simulink model "Advanced_Voter"  (R2018b)
settings: Solver=VariableStepAuto  StartTime=0.0  StopTime=10.0  RelTol=1e-3
settings Model: Creator=diepe  LastModifiedBy=diepe

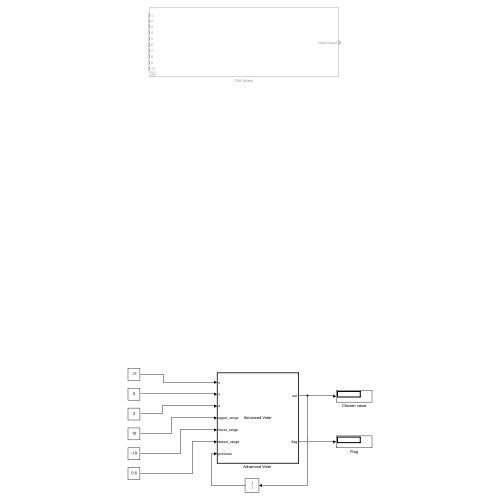
[thumbnail: Simulink's stored preview of the top-level diagram]
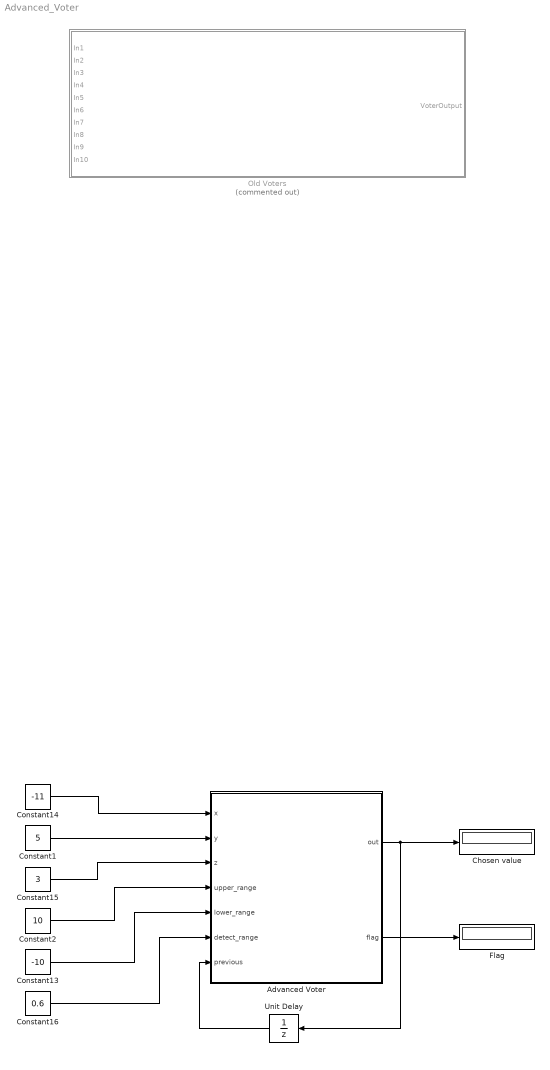
== system Advanced_Voter ==
  "Advanced Voter " : MATLAB Function  TreatAsAtomicUnit=on
  Chosen value : Display
  Constant1 : Constant  Value=5  OutDataTypeStr=double
  Constant13 : Constant  Value=-10  OutDataTypeStr=double
  Constant14 : Constant  Value=-11  OutDataTypeStr=double
  Constant15 : Constant  Value=3  OutDataTypeStr=double
  Constant16 : Constant  Value=0.6  OutDataTypeStr=double
  Constant2 : Constant  Value=10  OutDataTypeStr=double
  Flag : Display
  Old Voters : Subsystem  Commented=on
  Unit Delay : UnitDelay  SampleTime=-1  HasFrameUpgradeWarning=on
  wires:
  Unit Delay/1 -> "Advanced Voter "/7(previous)
  Constant2/1 -> "Advanced Voter "/4(upper_range)
  Constant14/1 -> "Advanced Voter "/1(x)
  Constant1/1 -> "Advanced Voter "/2(y)
  Constant13/1 -> "Advanced Voter "/5(lower_range)
  Constant15/1 -> "Advanced Voter "/3(z)
  Constant16/1 -> "Advanced Voter "/6(detect_range)
  "Advanced Voter "/2(flag) -> Flag/1
  "Advanced Voter "/1(out) -> Chosen value/1, Unit Delay/1

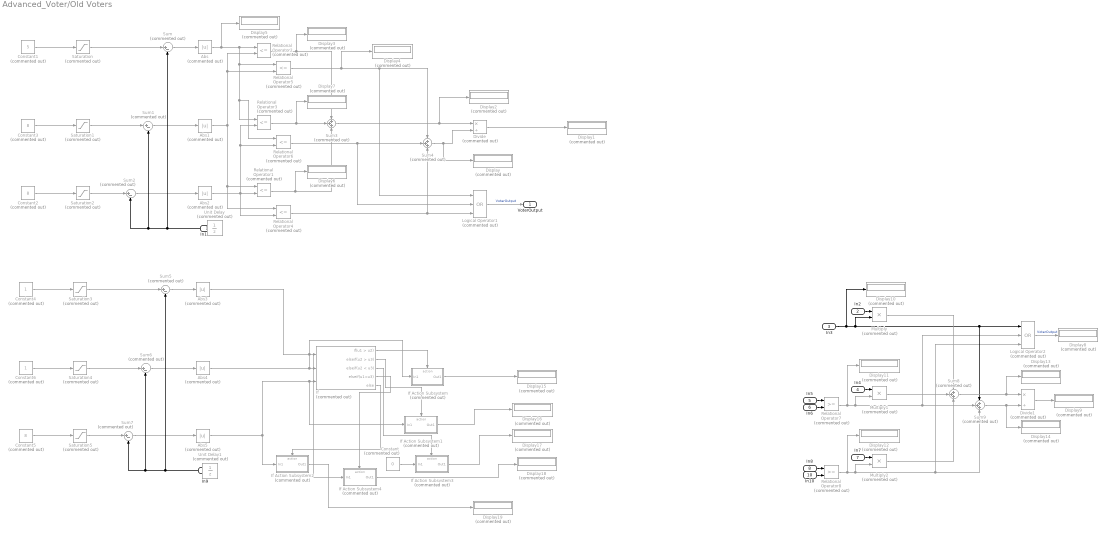
== system Advanced_Voter/Old Voters ==
  In1 : Inport
  In2 : Inport  Port=2
  In3 : Inport  Port=3
  In4 : Inport  Port=4
  In5 : Inport  Port=5
  In6 : Inport  Port=6
  In7 : Inport  Port=7
  In8 : Inport  Port=8
  In9 : Inport  Port=9
  In10 : Inport  Port=10
  Abs{,1..5} (6 alike) : Abs  Commented=on
  Constant : Constant  Commented=on  Value=0
  Constant1 : Constant  Commented=on  Value=5  OutDataTypeStr=int16
  Constant2 : Constant  Commented=on  Value=8  OutDataTypeStr=int16
  Constant3 : Constant  Commented=on  Value=8  OutDataTypeStr=int16
  Constant4 : Constant  Commented=on  OutDataTypeStr=int16
  Constant5 : Constant  Commented=on  Value=8  OutDataTypeStr=int16
  Constant6 : Constant  Commented=on  OutDataTypeStr=int16
  Display{,1..19} (20 alike) : Display  Commented=on
  Divide : Product  Commented=on  Inputs=*/
  Divide1 : Product  Commented=on  Inputs=*/
  If : If  Commented=on  NumInputs=3  IfExpression=u1 > u2  ElseIfExpressions=u2 > u3, u2 < u3, u1<u3
  If Action Subsystem : Subsystem  Commented=on  TreatAsAtomicUnit=on
  If Action Subsystem1 : Subsystem  Commented=on  TreatAsAtomicUnit=on
  If Action Subsystem2 : Subsystem  Commented=on  TreatAsAtomicUnit=on
  If Action Subsystem3 : Subsystem  Commented=on  TreatAsAtomicUnit=on
  If Action Subsystem4 : Subsystem  Commented=on  TreatAsAtomicUnit=on
  Logical Operator1 : Logic  Commented=on  Operator=OR  Inputs=3  AllPortsSameDT=off  OutDataTypeStr=boolean
  Logical Operator2 : Logic  Commented=on  Operator=OR  Inputs=3  AllPortsSameDT=off  OutDataTypeStr=boolean
  Multiply : Product  Commented=on
  Multiply1 : Product  Commented=on
  Multiply2 : Product  Commented=on
  Relational Operator1 : RelationalOperator  Commented=on  Operator=<=  RndMeth=Simplest
  Relational Operator{2,4..6} (4 alike) : RelationalOperator  Commented=on  Operator=<=  OutDataTypeStr=boolean  RndMeth=Simplest
  Relational Operator3 : RelationalOperator  Commented=on  Operator=<=  RndMeth=Simplest
  Relational Operator7 : RelationalOperator  Commented=on  OutDataTypeStr=boolean  RndMeth=Simplest
  Relational Operator8 : RelationalOperator  Commented=on  OutDataTypeStr=boolean  RndMeth=Simplest
  Saturation{,1..5} (6 alike) : Saturate  Commented=on  UpperLimit=10  LowerLimit=-10
  Sum{,1..2,5..7} (6 alike) : Sum  Commented=on  Inputs=|+-
  Sum{3..4,8..9} (4 alike) : Sum  Commented=on  Inputs=+++
  Unit Delay : UnitDelay  Commented=on  SampleTime=-1  HasFrameUpgradeWarning=on
  Unit Delay1 : UnitDelay  Commented=on  SampleTime=-1  HasFrameUpgradeWarning=on
  VoterOutput : Outport
  wires:
  Sum1/1 -> Abs1/1
  Abs3/1 -> If Action Subsystem4/1(In1), If/1
  Saturation/1 -> Sum/1
  Relational Operator8/1 -> Display12/1, Logical Operator2/3, Sum9/3, Multiply2/2
  Sum4/1 -> Display/1, Divide/2
  Relational Operator3/1 -> Display7/1, Sum3/2
  If Action Subsystem3/1(Out1) -> Display17/1
  Relational Operator7/1 -> Display11/1, Logical Operator2/2, Sum9/2, Multiply1/2
  Relational Operator1/1 -> Display6/1, Sum3/3
  Abs/1 -> Display5/1, Relational Operator5/1, Relational Operator6/1, Relational Operator3/1, Relational Operator2/1
  In3/1 -> Display10/1, Logical Operator2/1, Sum9/1, Multiply/2
  Relational Operator5/1 -> Display4/1, Sum4/1, Logical Operator1/1
  Abs1/1 -> Relational Operator4/1, Relational Operator1/1, Relational Operator5/2, Relational Operator2/2
  Sum5/1 -> Abs3/1
  Constant6/1 -> Saturation4/1
  Sum7/1 -> Abs5/1
  Sum9/1 -> Display14/1, Divide1/2
  Divide1/1 -> Display9/1
  Divide/1 -> Display1/1
  If Action Subsystem1/1(Out1) -> Display16/1
  Sum2/1 -> Abs2/1
  If/3 -> If Action Subsystem3/Action
  Saturation1/1 -> Sum1/1
  Sum/1 -> Abs/1
  Relational Operator2/1 -> Display3/1, Sum3/1
  Sum3/1 -> Display2/1, Divide/1
  Saturation4/1 -> Sum6/1
  Constant4/1 -> Saturation3/1
  Constant2/1 -> Saturation2/1
  If Action Subsystem4/1(Out1) -> Display18/1
  Constant3/1 -> Saturation1/1
  Abs4/1 -> If Action Subsystem/1(In1), If/2
  Relational Operator6/1 -> Sum4/2, Logical Operator1/2
  Sum6/1 -> Abs4/1
  In7/1 -> Multiply2/1
  Multiply/1 -> Sum8/1
  Saturation3/1 -> Sum5/1
  Multiply2/1 -> Sum8/3
  Abs2/1 -> Relational Operator6/2, Relational Operator3/2, Relational Operator4/2, Relational Operator1/2
  Sum8/1 -> Display13/1, Divide1/1
  In2/1 -> Multiply/1
  Constant5/1 -> Saturation5/1
  Logical Operator2/1 -> Display8/1  "VoterOutput"
  If/1 -> If Action Subsystem/Action
  If Action Subsystem2/1(Out1) -> Display19/1
  Saturation5/1 -> Sum7/1
  In1/1 -> Sum2/2, Sum1/2, Sum/2
  If/4 -> If Action Subsystem4/Action
  In8/1 -> Relational Operator8/1
  If/5 -> If Action Subsystem2/Action
  Multiply1/1 -> Sum8/2
  Abs5/1 -> If Action Subsystem2/1(In1), If Action Subsystem1/1(In1), If/3
  If Action Subsystem/1(Out1) -> Display15/1
  If/2 -> If Action Subsystem1/Action
  In9/1 -> Sum7/2, Sum6/2, Sum5/2
  Constant1/1 -> Saturation/1
  Constant/1 -> If Action Subsystem3/1(In1)
  In5/1 -> Relational Operator7/1
  Saturation2/1 -> Sum2/1
  Relational Operator4/1 -> Sum4/3, Logical Operator1/3
  In4/1 -> Multiply1/1
  Logical Operator1/1 -> VoterOutput/1  "VoterOutput"
  In10/1 -> Relational Operator8/2
  In6/1 -> Relational Operator7/2

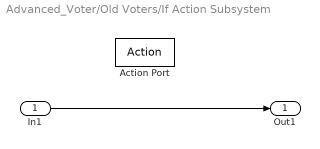
== system Advanced_Voter/Old Voters/If Action Subsystem ==
  In1 : Inport
  Action Port : ActionPort
  Out1 : Outport  VectorParamsAs1DForOutWhenUnconnected=off
  wires:
  In1/1 -> Out1/1

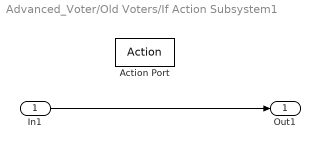
== system Advanced_Voter/Old Voters/If Action Subsystem1 ==
  In1 : Inport
  Action Port : ActionPort
  Out1 : Outport  VectorParamsAs1DForOutWhenUnconnected=off
  wires:
  In1/1 -> Out1/1

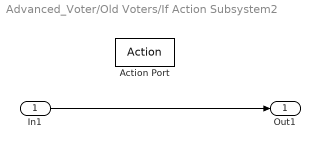
== system Advanced_Voter/Old Voters/If Action Subsystem2 ==
  In1 : Inport
  Action Port : ActionPort
  Out1 : Outport  VectorParamsAs1DForOutWhenUnconnected=off
  wires:
  In1/1 -> Out1/1

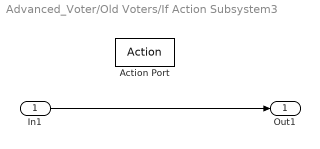
== system Advanced_Voter/Old Voters/If Action Subsystem3 ==
  In1 : Inport
  Action Port : ActionPort
  Out1 : Outport  VectorParamsAs1DForOutWhenUnconnected=off
  wires:
  In1/1 -> Out1/1

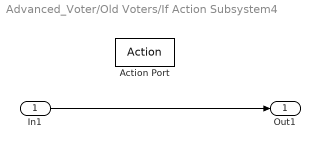
== system Advanced_Voter/Old Voters/If Action Subsystem4 ==
  In1 : Inport
  Action Port : ActionPort
  Out1 : Outport  VectorParamsAs1DForOutWhenUnconnected=off
  wires:
  In1/1 -> Out1/1

== matlab function Advanced_Voter/Advanced Voter  ==
  data: x input; y input; out output; z input; upper_range input; lower_range input; flag output; detect_range input; previous input
function [out, flag] = fcn(x,y,z,upper_range,lower_range, detect_range, previous)

% Distances are calculated between the values. Any negative value will be
% made positive
xy = abs(x-y);
xz = abs(x-z);
yz = abs(y-z);

% Determine which statements are true (statement,y,z)
sx = (x>upper_range) || (x<lower_range) || (isnan(x));
sy = (y>upper_range) || (y<lower_range) || (isnan(y));
sz = (z>upper_range) || (z<lower_range) || (isnan(z));

if sx == 1 && sy == 1 && sz == 1				% Every value is rejected
	% Previous output is taken
	out = previous;
	flag = 19;
elseif sx == 1 && sy == 1						% Value 'x' and 'y' are rejected by range or unknown
	% Only 'z'is eligable
	out = z;
	flag = 14;
elseif sx == 1 && sz == 1						% Value 'x' and 'z' are rejected by range or unknown
	% Only 'y' is eligable
	out = y;
	flag = 15;
elseif sy == 1 && sz == 1						% Value 'y' and ''z' are rejected by range or unknown
	% Only 'x'is eligable
	out = x;
	flag = 16;
elseif sx == 1									% Value 'x' is rejected by range or unknown
	% only 'yz' is eligable
	out = (y + z)/2;
	flag = 11;
elseif sy == 1									% Value 'y' is rejected by range or unknown
	% Only 'xz' is eligable
	out = (x + z)/2;
	flag = 12;
elseif sz == 1									% Value 'z' is rejected by range or unknown
	% Only 'xy' is eligable
	out = (x + y)/2;
	flag = 13;
else											% Nothing is rejected by range or unknown
	% The shortest distance is selected by the 'min' command. The selected
	% values are counted up and divided to get the mean. This value is
	% reported.
	if xy == min([xy xz yz])
		out = (x + y)/2;
	elseif xz == min([xy xz yz])
		out = (x + z)/2;
	else
		out = (y + z)/2;
	end
	flag = 10;
end

% Define the upper and lower detect range based on the chosen output
upper_detect_range = out * (1 + detect_range);
lower_detect_range = -(out * detect_range);

dx = (x>upper_detect_range) || (x<lower_detect_range);
dy = (y>upper_detect_range) || (y<lower_detect_range);
dz = (z>upper_detect_range) || (z<lower_detect_range);

if dx == 1 && dy == 1 && dz == 1
	flag = 19;
elseif dx == 1 && dy == 1
	flag = 14;
elseif dx == 1 && dz == 1
	flag = 15;
elseif dy == 1 && dz == 1
	flag = 16;
elseif dx == 1
	flag = 11;
elseif dy == 1
	flag = 12;
elseif dz == 1
	flag = 13;
else
	flag = 10;
end


end
